simulink model "Tarea_vacaciones"  (R2013a)
settings: Solver=ode45  StartTime=0.0  StopTime=10.0  RelTol=1e-3
libraries: powerlib x40, powerlib_meascontrol x10
settings Model: Creator=Miguel  LastModifiedBy=Miguel

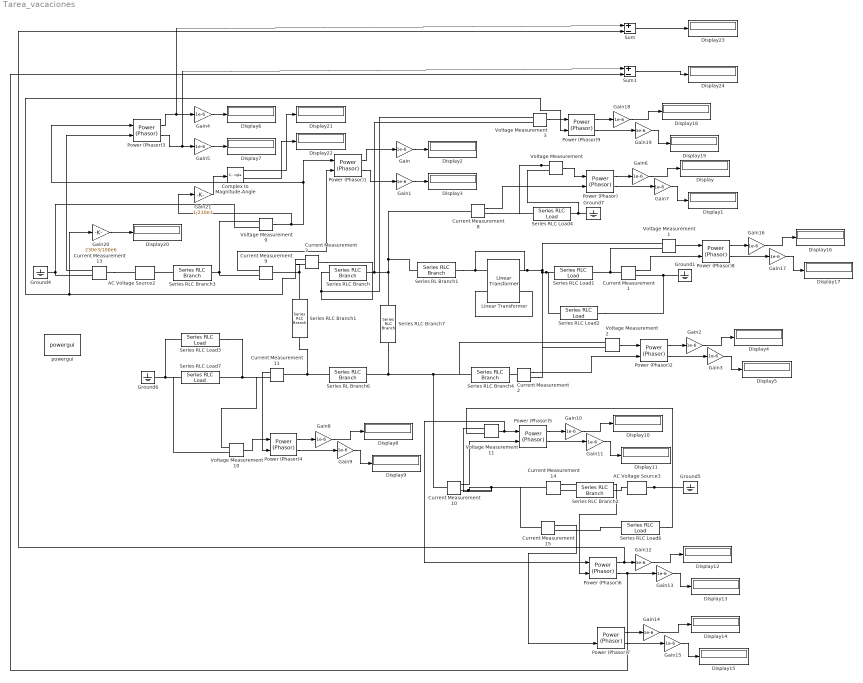
== system Tarea_vacaciones ==
  AC Voltage Source2 : powerlib/Electrical Sources/AC Voltage Source  Amplitude=1.01*230e3*sqrt(2)  Phase=0  Frequency=60  SampleTime=0  Measurements=None
  AC Voltage Source3 : powerlib/Electrical Sources/AC Voltage Source  Amplitude=1.0*sqrt(2)*230e3  Phase=-0.7528  Frequency=60  SampleTime=0  Measurements=None
  Complex to Magnitude-Angle : ComplexToMagnitudeAngle
  Current Measurement{1..3,8..11,13..15} (10 alike) : powerlib/Measurements/Current Measurement  PhasorSimulation=on  OutputType=Complex  PSBequivalent=0
  Display{,1..24} (25 alike) : Display
  Gain{,1..19} (20 alike) : Gain  Gain=1e-6
  Gain20 : Gain  Gain=230e3/100e6
  Gain21 : Gain  Gain=1/230e3
  Ground{1,4..7} (5 alike) : powerlib/Elements/Ground  LConnTagsString=a
  Linear Transformer : powerlib/Elements/Linear Transformer  LConnTagsString=a|b  RConnTagsString=A|B  UNITS=SI  NominalPower=[ 1000e6 60 ]  winding1=[0.9925*230e3 0 0.04/(2*pi*60)*230e3^2/100e6]  winding2=[0.9718*230e3 0 0]  ThreeWindings=off  winding3=[3.15e+05 0.7938 0.084225]  RmLm=[1.0805e+06 2866]  Measurements=Winding currents  DataType=on
  Power (Phasor){,1..9} (10 alike) : powerlib_meascontrol/Measurements/Power (Phasor)
  Series RL Branch1 : powerlib/Elements/Series RLC Branch  LConnTagsString=__new0  RConnTagsString=__new0  BranchType=L  Resistance=0.0118*230e3^2/100e6  Inductance=0.04/(2*pi*60)*230e3^2/100e6  SetiL0=off  InitialCurrent=0  Capacitance=1e-6  Setx0=off  InitialVoltage=0  Measurements=None
  Series RL Branch6 : powerlib/Elements/Series RLC Branch  LConnTagsString=__new0  RConnTagsString=__new0  BranchType=RL  Resistance=0.0118*230e3^2/100e6  Inductance=0.0529/(2*pi*60)*230e3^2/100e6  SetiL0=off  InitialCurrent=0  Capacitance=1e-6  Setx0=off  InitialVoltage=0  Measurements=None
  Series RLC Branch : powerlib/Elements/Series RLC Branch  LConnTagsString=__new0  RConnTagsString=__new0  BranchType=RL  Resistance=0.0108*230e3^2/100e6  Inductance=0.0649/(2*pi*60)*230e3^2/100e6  SetiL0=off  InitialCurrent=0  Capacitance=1e-6  Setx0=off  InitialVoltage=0  Measurements=None
  Series RLC Branch1 : powerlib/Elements/Series RLC Branch  LConnTagsString=__new0  RConnTagsString=__new0  BranchType=RL  Resistance=0.0235*230e3^2/100e6  Inductance=0.0941/(2*pi*60)*230e3^2/100e6  SetiL0=off  InitialCurrent=0  Capacitance=1e-6  Setx0=off  InitialVoltage=0  Measurements=None
  Series RLC Branch2 : powerlib/Elements/Series RLC Branch  LConnTagsString=__new0  RConnTagsString=__new0  BranchType=R  Resistance=1e-5  Inductance=1e-3  SetiL0=off  InitialCurrent=0  Capacitance=1e-6  Setx0=off  InitialVoltage=0  Measurements=None
  Series RLC Branch3 : powerlib/Elements/Series RLC Branch  LConnTagsString=__new0  RConnTagsString=__new0  BranchType=R  Resistance=1e-5  Inductance=1e-3  SetiL0=off  InitialCurrent=0  Capacitance=1e-6  Setx0=off  InitialVoltage=0  Measurements=None
  Series RLC Branch4 : powerlib/Elements/Series RLC Branch  LConnTagsString=__new0  RConnTagsString=__new0  BranchType=RL  Resistance=0.0147*230e3^2/100e6  Inductance=0.0588/(2*pi*60)*230e3^2/100e6  SetiL0=off  InitialCurrent=0  Capacitance=1e-6  Setx0=off  InitialVoltage=0  Measurements=None
  Series RLC Branch7 : powerlib/Elements/Series RLC Branch  LConnTagsString=__new0  RConnTagsString=__new0  BranchType=RL  Resistance=0.0118*230e3^2/100e6  Inductance=0.0471/(2*pi*60)*230e3^2/100e6  SetiL0=off  InitialCurrent=0  Capacitance=1e-6  Setx0=off  InitialVoltage=0  Measurements=None
  Series RLC Load1 : powerlib/Elements/Series RLC Load  LConnTagsString=a  RConnTagsString=__new0  NominalVoltage=0.9718*230e3  NominalFrequency=60  ActivePower=70e6  InductivePower=42e6  CapacitivePower=0  Setx0=off  InitialVoltage=0  SetiL0=off  InitialCurrent=0  Measurements=Branch current
  Series RLC Load2 : powerlib/Elements/Series RLC Load  LConnTagsString=a  RConnTagsString=__new0  NominalVoltage=0.9718*230e3  NominalFrequency=60  ActivePower=0  InductivePower=0  CapacitivePower=18e6  Setx0=off  InitialVoltage=0  SetiL0=off  InitialCurrent=0  Measurements=Branch current
  Series RLC Load3 : powerlib/Elements/Series RLC Load  LConnTagsString=a  RConnTagsString=__new0  NominalVoltage=0.9847*230e3  NominalFrequency=60  ActivePower=0  InductivePower=0  CapacitivePower=15e6  Setx0=off  InitialVoltage=0  SetiL0=off  InitialCurrent=0  Measurements=Branch current
  Series RLC Load4 : powerlib/Elements/Series RLC Load  LConnTagsString=a  RConnTagsString=__new0  NominalVoltage=0.9925*230e3  NominalFrequency=60  ActivePower=60e6  InductivePower=35e6  CapacitivePower=0  Setx0=off  InitialVoltage=0  SetiL0=off  InitialCurrent=0  Measurements=None
  Series RLC Load6 : powerlib/Elements/Series RLC Load  LConnTagsString=a  RConnTagsString=__new0  NominalVoltage=1.0*230e3  NominalFrequency=60  ActivePower=65e6  InductivePower=36e6  CapacitivePower=0  Setx0=off  InitialVoltage=0  SetiL0=off  InitialCurrent=0  Measurements=None
  Series RLC Load7 : powerlib/Elements/Series RLC Load  LConnTagsString=a  RConnTagsString=__new0  NominalVoltage=0.9847*230e3  NominalFrequency=60  ActivePower=80e6  InductivePower=50e6  CapacitivePower=0  Setx0=off  InitialVoltage=0  SetiL0=off  InitialCurrent=0  Measurements=Branch current
  Sum : Sum  Inputs=|+-
  Sum1 : Sum  Inputs=|+-
  Voltage Measurement{,1..3,9..11} (7 alike) : powerlib/Measurements/Voltage Measurement  PhasorSimulation=on  OutputType=Complex  PSBequivalent=0
  powergui : powerlib/powergui  Priority=1  SimulationMode=Phasor  SolverType=Tustin  SampleTime=50e-6  frequency=60  SPID=off  DisableSnubberDevices=off  DisableRonSwitches=off  DisableVfSwitches=off  SwTol=0  Interpol=off  DisplayEquations=off  frequencyindice=60  Pbase=100e6  ErrMax=1e-4  Iterations=50  UnitsV=kV  UnitsW=MW  FunctionMessages=off  echomessages=off  HookPort=off  EnableUseOfTLC=off  x0status=blocks  RestoreLinks=warning  ResistiveCurrentMeasurement=off  Frange=[0:2:500]  Ylog=off  Xlog=on  ShowGrid=off  save=off  variable=ZData  ZoomFFT=off  StartTime=0.0  cycles=1  DisplayStyle=1  fundamental=60  FreqAxis=off  MaxFrequency=1000  frequencyindicesteady=1  RmsSteady=2  display=off  Ts=0  methode=off
  wires:
  Power (Phasor)/1 -> Gain6/1
  Power (Phasor)/2 -> Gain7/1
  Voltage Measurement/1 -> Power (Phasor)/1
  Current Measurement8/1 -> Power (Phasor)/2
  Power (Phasor)1/1 -> Gain/1
  Power (Phasor)1/2 -> Gain1/1
  Current Measurement9/1 -> Power (Phasor)1/2
  Gain1/1 -> Display3/1
  Gain/1 -> Display2/1
  Power (Phasor)3/1 -> Sum/1, Gain4/1
  Power (Phasor)3/2 -> Sum1/1, Gain5/1
  Gain5/1 -> Display7/1
  Gain4/1 -> Display6/1
  Current Measurement13/1 -> Power (Phasor)3/2
  Gain6/1 -> Display/1
  Gain7/1 -> Display1/1
  Power (Phasor)4/1 -> Gain8/1
  Power (Phasor)4/2 -> Gain9/1
  Voltage Measurement10/1 -> Power (Phasor)4/1
  Current Measurement11/1 -> Power (Phasor)4/2
  Gain8/1 -> Display8/1
  Gain9/1 -> Display9/1
  Power (Phasor)5/2 -> Gain11/1
  Gain10/1 -> Display10/1
  Gain11/1 -> Display11/1
  Power (Phasor)6/1 -> Sum/2, Gain12/1
  Power (Phasor)6/2 -> Sum1/2, Gain13/1
  Gain12/1 -> Display12/1
  Gain13/1 -> Display13/1
  Power (Phasor)7/1 -> Gain14/1
  Power (Phasor)7/2 -> Gain15/1
  Voltage Measurement11/1 -> Power (Phasor)6/1, Power (Phasor)5/1
  Gain14/1 -> Display14/1
  Gain15/1 -> Display15/1
  Current Measurement10/1 -> Power (Phasor)5/2
  Current Measurement14/1 -> Power (Phasor)6/2
  Current Measurement15/1 -> Power (Phasor)7/2
  Power (Phasor)8/1 -> Gain16/1
  Power (Phasor)8/2 -> Gain17/1
  Gain16/1 -> Display16/1
  Gain17/1 -> Display17/1
  Voltage Measurement1/1 -> Power (Phasor)8/1
  Current Measurement1/1 -> Power (Phasor)8/2
  Power (Phasor)2/1 -> Gain2/1
  Power (Phasor)2/2 -> Gain3/1
  Gain2/1 -> Display4/1
  Gain3/1 -> Display5/1
  Voltage Measurement2/1 -> Power (Phasor)2/1
  Current Measurement2/1 -> Power (Phasor)2/2
  Power (Phasor)9/1 -> Gain18/1
  Power (Phasor)9/2 -> Gain19/1
  Gain18/1 -> Display18/1
  Gain19/1 -> Display19/1
  Voltage Measurement3/1 -> Power (Phasor)9/1
  Current Measurement3/1 -> Gain20/1, Power (Phasor)9/2
  Gain20/1 -> Display20/1
  Voltage Measurement9/1 -> Gain21/1, Power (Phasor)1/1, Power (Phasor)3/1
  Gain21/1 -> Complex to Magnitude-Angle/1
  Complex to Magnitude-Angle/1 -> Display21/1
  Complex to Magnitude-Angle/2 -> Display22/1
  Sum1/1 -> Display24/1
  Sum/1 -> Display23/1
  Power (Phasor)5/1 -> Gain10/1
  connections:
  Ground4/LConn1 -- Voltage Measurement9/LConn2 -- Current Measurement13/RConn1
  Series RLC Branch1/RConn1 -- Current Measurement11/LConn1 -- Series RL Branch6/LConn1
  Voltage Measurement/LConn1 -- Series RLC Load4/LConn1 -- Current Measurement8/RConn1
  Current Measurement10/LConn1 -- Voltage Measurement2/LConn1 -- Series RLC Branch4/LConn1 -- Series RLC Branch7/RConn1 -- Series RL Branch6/RConn1
  AC Voltage Source3/LConn1 -- Ground5/LConn1 -- Voltage Measurement11/LConn2 -- Series RLC Load6/RConn1
  Series RLC Load7/RConn1 -- Voltage Measurement10/LConn2 -- Series RLC Load3/LConn1 -- Ground6/LConn1
  Series RLC Load4/RConn1 -- Ground7/LConn1 -- Voltage Measurement/LConn2
  Series RLC Branch1/LConn1 -- Current Measurement3/RConn1 -- Current Measurement9/LConn1
  Current Measurement11/RConn1 -- Voltage Measurement10/LConn1 -- Series RLC Load3/RConn1 -- Series RLC Load7/LConn1
  Current Measurement10/RConn1 -- Voltage Measurement11/LConn1 -- Current Measurement15/LConn1 -- Current Measurement14/LConn1
  Current Measurement9/RConn1 -- Voltage Measurement9/LConn1 -- Series RLC Branch3/RConn1
  Current Measurement13/LConn1 -- AC Voltage Source2/LConn1
  Series RLC Load6/LConn1 -- Current Measurement15/RConn1
  Series RLC Branch2/LConn1 -- Current Measurement14/RConn1
  Series RLC Branch2/RConn1 -- AC Voltage Source3/RConn1
  Current Measurement1/LConn1 -- Voltage Measurement1/LConn2 -- Series RLC Load1/RConn1
  Ground1/LConn1 -- Series RLC Load2/RConn1 -- Current Measurement1/RConn1
  Current Measurement2/LConn1 -- Series RLC Branch4/RConn1
  Current Measurement3/LConn1 -- Series RLC Branch/LConn1 -- Voltage Measurement3/LConn1
  Linear Transformer/LConn2 -- Linear Transformer/RConn2
  Series RLC Branch3/LConn1 -- AC Voltage Source2/RConn1
  Series RL Branch1/RConn1 -- Series RLC Load1/LConn1 -- Series RLC Load2/LConn1 -- Current Measurement2/RConn1 -- Voltage Measurement2/LConn2 -- Voltage Measurement1/LConn1 -- Linear Transformer/RConn1 -- Linear Transformer/LConn1
  Current Measurement8/LConn1 -- Series RL Branch1/LConn1 -- Series RLC Branch7/LConn1 -- Voltage Measurement3/LConn2 -- Series RLC Branch/RConn1
